simulink model "Crane3D_DevDriv_READY"  (R2015a)
settings: Solver=ode4  StartTime=0.0  StopTime=Inf  FixedStep=0.001  RelTol=1e-3
undefined symbols (not defined in the file or in its folder): alphaXscale, alphaYscale, Crane3D_RangeBit, Crane3D_ScaleCoeff, eXscale, eYscale, kX, kY
undefined symbols (not defined in the file): RTDAC4PCIBaseAddress
settings Model: SimulationMode=external  CovSFcnEnable=off  ExtModeTrigMode=oneshot  ExtModeTrigDuration=10000  Creator=The MathWorks Inc.  LastModifiedBy=Student
settings DataIOCC: Decimation=10  LimitDataPoints=off  SignalLoggingSaveFormat=ModelDataLogs  SignalLoggingName=logsOut
settings OptimizationCC: ExpressionDepthLimit=2147483647  InitFltsAndDblsToZero=on  EfficientMapNaN2IntZero=off
settings DebuggingCC: UnderspecifiedInitializationDetection=Classic  MergeDetectMultiDrivingBlocksExec=none  SignalResolutionControl=TryResolveAllWithWarning  FcnCallInpInsideContextMsg=UseLocalSettings  StateNameClashWarn=warning
settings HardwareCC: ProdBitPerLong=64  ProdBitPerPointer=64  ProdIntDivRoundTo=Zero  ProdEndianess=LittleEndian  ProdWordSize=64  ProdHWDeviceType=Intel->x86-64  TargetBitPerLong=64  TargetBitPerPointer=64  TargetIntDivRoundTo=Zero  TargetEndianess=LittleEndian  TargetWordSize=64  TargetHWDeviceType=Intel->x86-64
settings RTWCC: SystemTargetFile=rtwin.tlc  TemplateMakefile=rtwin.tmf  Description=Real-Time Windows Target
settings RTWinTargetCC: TargetPreCompLibLocation=C:\Program Files\MATLAB\R2015aSP1\toolbox\sldrt\lib\win64

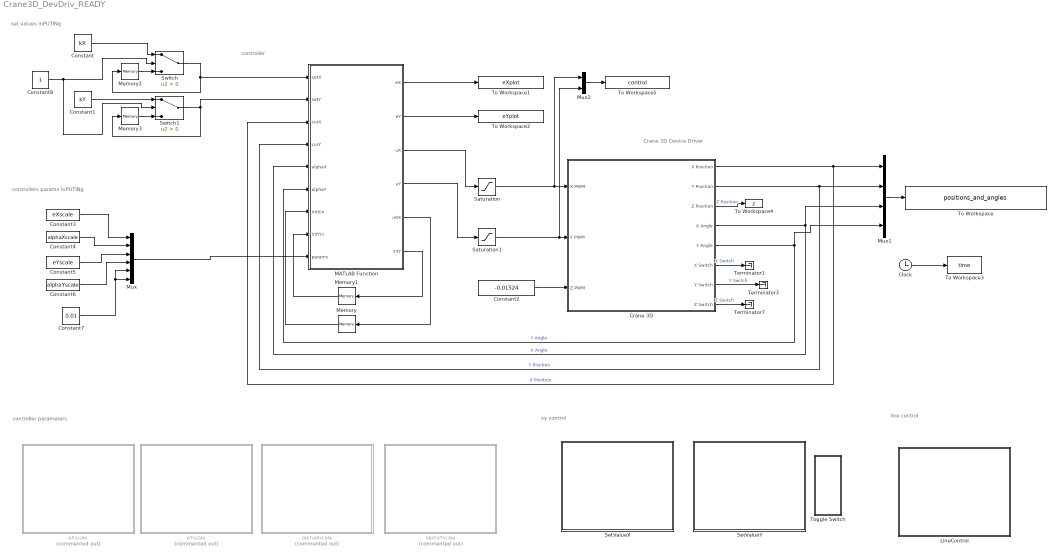
== system Crane3D_DevDriv_READY ==
  note: controller
  note: Crane 3D Device Driver
  note: set values inPUTINg
  note: controllers params inPUTINg
  note: line control
  note: xy control
  note: controller parameters
  Clock : Clock
  Constant : Constant  Value=kX
  Constant1 : Constant  Value=kY
  Constant2 : Constant  Value=-0.01524
  Constant3 : Constant  Value=eXscale
  Constant4 : Constant  Value=alphaXscale
  Constant5 : Constant  Value=eYscale
  Constant6 : Constant  Value=alphaYscale
  Constant7 : Constant  Value=0.01
  Constant8 : Constant
  Crane 3D : Subsystem  mask{BaseAddress=RTDAC4PCIBaseAddress, T0=0.001}
      mask prompts: BaseAddress "Base Address:"; T0 "Samping Period:"
      mask Display: image(imread('crane.jpeg'))
  LineControl : Subsystem  DialogController=hmiCreateDDGDialog  IsWebBlock=on  mask(MathWorksWebBlock){webBlockId=fac2dc05-0e7c-4443-aafa-0c4be83aaef0, webBlockType=continuousknob, ShowInLibBrowser=on, ShowInitialText=on, HMISrcModelName=Crane3D_DevDriv_READY}
      mask prompts: webBlockId "WebBlock Id"; webBlockType "WebBlock Type"; HMISrcModelName "Source Model"
      mask Help: helpview([docroot '/mapfiles/simulink.map'], 'hmi_knob')
      mask Display:
      | if strcmp(get_param(bdroot(gcb),'BlockDiagramType'), 'library')
      |     image([(matlabroot) '/toolbox/simulink/hmi/icons/ContinuousKnob.png']);
      | end
  MATLAB Function : MATLAB Function  TreatAsAtomicUnit=on
  Memory{,1..3} (4 alike) : Memory
  Mux : Mux  Inputs=6
  Mux1 : Mux
  Mux2 : Mux  Inputs=2
  Saturation : Saturate  UpperLimit=0.4  LowerLimit=-0.4
  Saturation1 : Saturate  UpperLimit=0.4  LowerLimit=-0.4
  SetValueX : Subsystem  DialogController=hmiCreateDDGDialog  IsWebBlock=on  mask(MathWorksWebBlock){webBlockId=89ff67ae-b140-41c3-b09d-3fb2d6446b16, webBlockType=continuousknob, ShowInLibBrowser=on, ShowInitialText=on, HMISrcModelName=Crane3D_DevDriv_READY}
      mask prompts: webBlockId "WebBlock Id"; webBlockType "WebBlock Type"; HMISrcModelName "Source Model"
      mask Help: helpview([docroot '/mapfiles/simulink.map'], 'hmi_knob')
      mask Display:
      | if strcmp(get_param(bdroot(gcb),'BlockDiagramType'), 'library')
      |     image([(matlabroot) '/toolbox/simulink/hmi/icons/ContinuousKnob.png']);
      | end
  "SetValueY " : Subsystem  DialogController=hmiCreateDDGDialog  IsWebBlock=on  mask(MathWorksWebBlock){webBlockId=c2e642d5-e8be-48aa-bd7f-80d5e0063407, webBlockType=continuousknob, ShowInLibBrowser=on, ShowInitialText=on, HMISrcModelName=Crane3D_DevDriv_READY}
      mask prompts: webBlockId "WebBlock Id"; webBlockType "WebBlock Type"; HMISrcModelName "Source Model"
      mask Help: helpview([docroot '/mapfiles/simulink.map'], 'hmi_knob')
      mask Display:
      | if strcmp(get_param(bdroot(gcb),'BlockDiagramType'), 'library')
      |     image([(matlabroot) '/toolbox/simulink/hmi/icons/ContinuousKnob.png']);
      | end
  Switch : Switch  Criteria=u2 > Threshold
  Switch1 : Switch  Criteria=u2 > Threshold
  Terminator1 : Terminator
  Terminator3 : Terminator
  Terminator7 : Terminator
  To Workspace : ToWorkspace  VariableName=positions_and_angles  SampleTime=-1
  To Workspace1 : ToWorkspace  VariableName=eXplot  SampleTime=-1
  To Workspace2 : ToWorkspace  VariableName=eYplot  SampleTime=-1
  To Workspace3 : ToWorkspace  VariableName=time  SampleTime=-1
  To Workspace4 : ToWorkspace  VariableName=z  SampleTime=-1
  To Workspace5 : ToWorkspace  VariableName=control  SampleTime=-1
  Toggle Switch : Subsystem  DialogController=hmiCreateDDGDialog  IsWebBlock=on  mask(MathWorksWebBlock){webBlockId=800a7fb0-11df-43e5-8f6f-d8a653a38972, webBlockType=toggleswitch, ShowInLibBrowser=on, ShowInitialText=on, HMISrcModelName=Crane3D_DevDriv_READY}
      mask prompts: webBlockId "WebBlock Id"; webBlockType "WebBlock Type"; HMISrcModelName "Source Model"
      mask Help: helpview([docroot '/mapfiles/simulink.map'], 'hmi_toggle_switch')
      mask Display:
      | if strcmp(get_param(bdroot(gcb),'BlockDiagramType'), 'library')
      |     image([(matlabroot) '/toolbox/simulink/hmi/icons/ToggleSwitch.png']);
      | end
  alphaXscale : Subsystem  Commented=on  DialogController=hmiCreateDDGDialog  IsWebBlock=on  mask(MathWorksWebBlock){webBlockId=5c22c07c-1326-4956-b101-402927ca42f7, webBlockType=continuousknob, ShowInLibBrowser=on, ShowInitialText=on, HMISrcModelName=Crane3D_DevDriv_READY}
      mask prompts: webBlockId "WebBlock Id"; webBlockType "WebBlock Type"; HMISrcModelName "Source Model"
      mask Help: helpview([docroot '/mapfiles/simulink.map'], 'hmi_knob')
      mask Display:
      | if strcmp(get_param(bdroot(gcb),'BlockDiagramType'), 'library')
      |     image([(matlabroot) '/toolbox/simulink/hmi/icons/ContinuousKnob.png']);
      | end
  alphaYscale : Subsystem  Commented=on  DialogController=hmiCreateDDGDialog  IsWebBlock=on  mask(MathWorksWebBlock){webBlockId=33cac2b1-8caf-4bd8-9ba1-d42b720b6015, webBlockType=continuousknob, ShowInLibBrowser=on, ShowInitialText=on, HMISrcModelName=Crane3D_DevDriv_READY}
      mask prompts: webBlockId "WebBlock Id"; webBlockType "WebBlock Type"; HMISrcModelName "Source Model"
      mask Help: helpview([docroot '/mapfiles/simulink.map'], 'hmi_knob')
      mask Display:
      | if strcmp(get_param(bdroot(gcb),'BlockDiagramType'), 'library')
      |     image([(matlabroot) '/toolbox/simulink/hmi/icons/ContinuousKnob.png']);
      | end
  "eXscale " : Subsystem  Commented=on  DialogController=hmiCreateDDGDialog  IsWebBlock=on  mask(MathWorksWebBlock){webBlockId=bf9c4a83-d73f-47d8-b533-9092dac72cb6, webBlockType=continuousknob, ShowInLibBrowser=on, ShowInitialText=on, HMISrcModelName=Crane3D_DevDriv_READY}
      mask prompts: webBlockId "WebBlock Id"; webBlockType "WebBlock Type"; HMISrcModelName "Source Model"
      mask Help: helpview([docroot '/mapfiles/simulink.map'], 'hmi_knob')
      mask Display:
      | if strcmp(get_param(bdroot(gcb),'BlockDiagramType'), 'library')
      |     image([(matlabroot) '/toolbox/simulink/hmi/icons/ContinuousKnob.png']);
      | end
  eYscale : Subsystem  Commented=on  DialogController=hmiCreateDDGDialog  IsWebBlock=on  mask(MathWorksWebBlock){webBlockId=03d0d190-e749-4b18-a62c-b15af9981338, webBlockType=continuousknob, ShowInLibBrowser=on, ShowInitialText=on, HMISrcModelName=Crane3D_DevDriv_READY}
      mask prompts: webBlockId "WebBlock Id"; webBlockType "WebBlock Type"; HMISrcModelName "Source Model"
      mask Help: helpview([docroot '/mapfiles/simulink.map'], 'hmi_knob')
      mask Display:
      | if strcmp(get_param(bdroot(gcb),'BlockDiagramType'), 'library')
      |     image([(matlabroot) '/toolbox/simulink/hmi/icons/ContinuousKnob.png']);
      | end
  wires:
  Crane 3D/8(Z Switch) -> Terminator7/1  "Z Switch"
  Crane 3D/1(X Position) -> MATLAB Function/3(curX), Mux1/1  "X Position"
  Crane 3D/2(Y Position) -> MATLAB Function/4(curY), Mux1/2  "Y Position"
  Crane 3D/3(Z Position) -> To Workspace4/1  "Z Position"
  Crane 3D/4(X Angle) -> Mux1/3, MATLAB Function/5(alphaX)  "X Angle"
  Crane 3D/5(Y Angle) -> Mux1/4, MATLAB Function/6(alphaY)  "Y Angle"
  Crane 3D/6(X Switch) -> Terminator1/1  "X Switch"
  Crane 3D/7(Y Switch) -> Terminator3/1  "Y Switch"
  Mux1/1 -> To Workspace/1
  Constant2/1 -> Crane 3D/3(Z PWM)
  MATLAB Function/2(eY) -> To Workspace2/1
  MATLAB Function/1(eX) -> To Workspace1/1
  MATLAB Function/5(intX) -> Memory/1
  MATLAB Function/6(intY) -> Memory1/1
  Clock/1 -> To Workspace3/1
  MATLAB Function/3(uX) -> Saturation/1
  MATLAB Function/4(uY) -> Saturation1/1
  Saturation1/1 -> Mux2/2, Crane 3D/2(Y PWM)
  Saturation/1 -> Mux2/1, Crane 3D/1(X PWM)
  Memory1/1 -> MATLAB Function/8(intYin)
  Memory/1 -> MATLAB Function/7(intXin)
  Switch/1 -> Memory2/1, MATLAB Function/1(setX)
  Constant/1 -> Switch/1
  Switch1/1 -> MATLAB Function/2(setY), Memory3/1
  Constant1/1 -> Switch1/1
  Memory2/1 -> Switch/3
  Memory3/1 -> Switch1/3
  Constant8/1 -> Switch1/2, Switch/2
  Mux/1 -> MATLAB Function/9(params)
  Constant3/1 -> Mux/1
  Constant4/1 -> Mux/2
  Constant5/1 -> Mux/3
  Constant6/1 -> Mux/4
  Constant7/1 -> Mux/5, Mux/6
  Mux2/1 -> To Workspace5/1

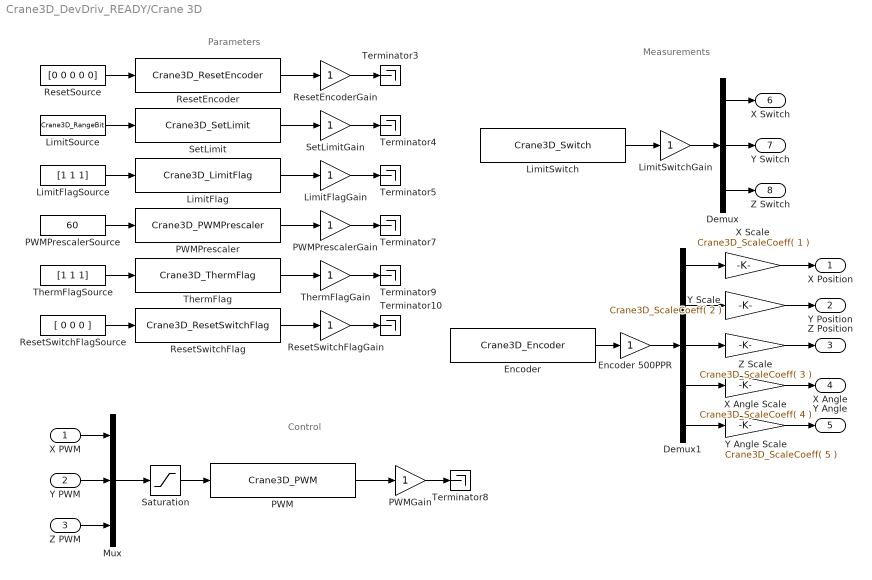
== system Crane3D_DevDriv_READY/Crane 3D ==
  note: Measurements
  note: Control
  note: Parameters
  X PWM : Inport
  Y PWM : Inport  Port=2
  Z PWM : Inport  Port=3
  Demux : Demux  Outputs=3
  Demux1 : Demux  Outputs=5
  Encoder : S-Function  FunctionName=Crane3D_Encoder  Parameters=BaseAddress, T0
  Encoder 500PPR : Gain  SaturateOnIntegerOverflow=on  OutDataTypeStr=Inherit: Same as input  ParamDataTypeStr=Inherit: Same as input
  LimitFlag : S-Function  FunctionName=Crane3D_LimitFlag  Parameters=BaseAddress, T0
  LimitFlagGain : Gain  SaturateOnIntegerOverflow=on  OutDataTypeStr=Inherit: Same as input  ParamDataTypeStr=Inherit: Same as input
  LimitFlagSource : Constant  Value=[1 1 1]
  LimitSource : Constant  Value=Crane3D_RangeBit
  LimitSwitch : S-Function  FunctionName=Crane3D_Switch  Parameters=BaseAddress, T0
  LimitSwitchGain : Gain  SaturateOnIntegerOverflow=on  OutDataTypeStr=Inherit: Same as input  ParamDataTypeStr=Inherit: Same as input
  Mux : Mux  Inputs=3
  PWM : S-Function  FunctionName=Crane3D_PWM  Parameters=BaseAddress, T0
  PWMGain : Gain  SaturateOnIntegerOverflow=on  OutDataTypeStr=Inherit: Same as input  ParamDataTypeStr=Inherit: Same as input
  PWMPrescaler : S-Function  FunctionName=Crane3D_PWMPrescaler  Parameters=BaseAddress, T0
  PWMPrescalerGain : Gain  SaturateOnIntegerOverflow=on  OutDataTypeStr=Inherit: Same as input  ParamDataTypeStr=Inherit: Same as input
  PWMPrescalerSource : Constant  Value=60
  ResetEncoder : S-Function  FunctionName=Crane3D_ResetEncoder  Parameters=BaseAddress, T0
  ResetEncoderGain : Gain  SaturateOnIntegerOverflow=on  OutDataTypeStr=Inherit: Same as input  ParamDataTypeStr=Inherit: Same as input
  ResetSource : Constant  Value=[0 0 0 0 0]
  "ResetSwitchFlag " : S-Function  FunctionName=Crane3D_ResetSwitchFlag  Parameters=BaseAddress, T0
  ResetSwitchFlagGain : Gain  SaturateOnIntegerOverflow=on  OutDataTypeStr=Inherit: Same as input  ParamDataTypeStr=Inherit: Same as input
  ResetSwitchFlagSource : Constant  Value=[ 0 0 0 ]
  Saturation : Saturate  UpperLimit=1  LowerLimit=-1
  SetLimit : S-Function  FunctionName=Crane3D_SetLimit  Parameters=BaseAddress, T0
  SetLimitGain : Gain  SaturateOnIntegerOverflow=on  OutDataTypeStr=Inherit: Same as input  ParamDataTypeStr=Inherit: Same as input
  Terminator{3..5,7..10} (7 alike) : Terminator
  "ThermFlag " : S-Function  FunctionName=Crane3D_ThermFlag  Parameters=BaseAddress, T0
  ThermFlagGain : Gain  SaturateOnIntegerOverflow=on  OutDataTypeStr=Inherit: Same as input  ParamDataTypeStr=Inherit: Same as input
  ThermFlagSource : Constant  Value=[1 1 1]
  X Angle Scale : Gain  Gain=Crane3D_ScaleCoeff( 4 )  OutDataTypeStr=Inherit: Same as input  ParamDataTypeStr=Inherit: Same as input
  X Scale : Gain  Gain=Crane3D_ScaleCoeff( 1 )  OutDataTypeStr=Inherit: Same as input  ParamDataTypeStr=Inherit: Same as input
  Y Angle Scale : Gain  Gain=Crane3D_ScaleCoeff( 5 )  OutDataTypeStr=Inherit: Same as input  ParamDataTypeStr=Inherit: Same as input
  Y Scale : Gain  Gain=Crane3D_ScaleCoeff( 2 )  OutDataTypeStr=Inherit: Same as input  ParamDataTypeStr=Inherit: Same as input
  Z Scale : Gain  Gain=Crane3D_ScaleCoeff( 3 )  OutDataTypeStr=Inherit: Same as input  ParamDataTypeStr=Inherit: Same as input
  X Position : Outport  InitialOutput=0
  Y Position : Outport  Port=2  InitialOutput=0
  Z Position : Outport  Port=3  InitialOutput=0
  X Angle : Outport  Port=4  InitialOutput=0
  Y Angle : Outport  Port=5  InitialOutput=0
  X Switch : Outport  Port=6  InitialOutput=0
  Y Switch : Outport  Port=7  InitialOutput=0
  Z Switch : Outport  Port=8  InitialOutput=0
  wires:
  Demux1/1 -> X Scale/1
  Demux1/2 -> Y Scale/1
  Demux1/3 -> Z Scale/1
  Demux1/4 -> X Angle Scale/1
  Demux1/5 -> Y Angle Scale/1
  X Angle Scale/1 -> X Angle/1
  Y Angle Scale/1 -> Y Angle/1
  Y Scale/1 -> Y Position/1
  X Scale/1 -> X Position/1
  Z Scale/1 -> Z Position/1
  Demux/3 -> Z Switch/1
  Demux/2 -> Y Switch/1
  Demux/1 -> X Switch/1
  LimitSwitchGain/1 -> Demux/1
  LimitSwitch/1 -> LimitSwitchGain/1
  X PWM/1 -> Mux/1
  Y PWM/1 -> Mux/2
  Z PWM/1 -> Mux/3
  ResetSwitchFlagGain/1 -> Terminator10/1
  ThermFlagGain/1 -> Terminator9/1
  PWMPrescalerGain/1 -> Terminator7/1
  LimitFlagGain/1 -> Terminator5/1
  SetLimitGain/1 -> Terminator4/1
  ResetEncoderGain/1 -> Terminator3/1
  ResetSwitchFlagSource/1 -> "ResetSwitchFlag "/1
  ThermFlagSource/1 -> "ThermFlag "/1
  PWMPrescalerSource/1 -> PWMPrescaler/1
  LimitFlagSource/1 -> LimitFlag/1
  LimitSource/1 -> SetLimit/1
  ResetSource/1 -> ResetEncoder/1
  "ResetSwitchFlag "/1 -> ResetSwitchFlagGain/1
  "ThermFlag "/1 -> ThermFlagGain/1
  PWMPrescaler/1 -> PWMPrescalerGain/1
  LimitFlag/1 -> LimitFlagGain/1
  SetLimit/1 -> SetLimitGain/1
  ResetEncoder/1 -> ResetEncoderGain/1
  PWMGain/1 -> Terminator8/1
  PWM/1 -> PWMGain/1
  Mux/1 -> Saturation/1
  Saturation/1 -> PWM/1
  Encoder/1 -> Encoder 500PPR/1
  Encoder 500PPR/1 -> Demux1/1

== system Crane3D_DevDriv_READY/LineControl ==

== system Crane3D_DevDriv_READY/SetValueX ==

== system Crane3D_DevDriv_READY/SetValueY  ==

== system Crane3D_DevDriv_READY/Toggle Switch ==

== system Crane3D_DevDriv_READY/alphaXscale ==

== system Crane3D_DevDriv_READY/alphaYscale ==

== system Crane3D_DevDriv_READY/eXscale  ==

== system Crane3D_DevDriv_READY/eYscale ==

== matlab function Crane3D_DevDriv_READY/MATLAB Function ==
  data: setX input; setY input; curX input; curY input; alphaX input; alphaY input; intXin input; intYin input; eX output; eY output; uX output; uY output; intX output; intY output; params input
function [ eX, eY, uX, uY, intX, intY ] = fcn(setX, setY, curX, curY, alphaX, alphaY, intXin, intYin, params)
%#codegen

dt = 0.001;

eX = setX - curX;
eY = setY - curY;

intX = intXin + eX * dt;
intY = intYin + eY * dt;

uX = params(1) * eX + params(2) * alphaX + params(5) * intX;
uY = params(3) * eY + params(4) * alphaY + params(6) * intY;
